simulink library "lib_energy_storage"  (Simulink 7.9)
settings: Solver=ode45  SolverMode=SingleTasking  StartTime=0.0  StopTime=10.0  RelTol=1e-3
undefined symbols (not defined in the file or in its folder): air_cp, amb_tmp, cyc_mph, enable_stop, ess_cap, ess_cap_scale, ess_cb, ess_cc, ess_coulombic_eff, ess_init_soc, ess_max_ah_cap, ess_max_p, ess_max_p_soc, ess_max_soc, ess_max_volts, ess_min_soc, ess_min_volts, ess_MMi, ess_MMo, ess_mod_airflow, ess_mod_cp, ess_mod_cpm, ess_mod_init_tmp, ess_module_mass, ess_module_num, ess_on, ess_parallel_mod_num, ess_r, ess_r_chg, ess_r_dis, ess_rc, ess_re, ess_res_scale_coef, ess_res_scale_fun, ess_rt, ess_set_tmp, ess_soc, ess_th_calc, ess_th_res, ess_th_res_off, ess_th_res_on, ess_tmp, ess_voc, fund_byu, fund_byuop, mc_min_volts, saber_air_temp, Saber_Battery_IO_File, saber_init_soc, saber_init_temp, saber_init_voc, saber_k_cb, saber_k_cc, saber_k_rc, saber_k_re, saber_k_rt, saber_k_soc, t_soc, time_step
libraries: lib_energy_storage x3
(part 3 of 3)

== system lib_energy_storage/Ess Choices/energy storage <ess> optima fundamental model/ess tmp/Tair,ave ==
  Qess_case : Inport
  Enable : EnablePort  StatesWhenEnabling=reset
  Block NOTES : Subsystem
      mask Display: disp('Block\nNOTES')
  Tamb-(Q/mcp)/2 : Fcn  Expr=amb_tmp - (u(1)/(ess_mod_airflow*air_cp))/2
  do ex calcs?1 : Constant  Value=ess_th_res_on
  Tair_ave : Outport  OutputWhenDisabled=reset  InitialOutput=amb_tmp
  Th Res : Outport  Port=2  OutputWhenDisabled=reset  InitialOutput=ess_th_res_off
  wires:
  do ex calcs?1/1 -> Th Res/1
  Qess_case/1 -> Tamb-(Q/mcp)/2/1
  Tamb-(Q/mcp)/2/1 -> Tair_ave/1

== system lib_energy_storage/Ess Choices/Ultracapacitor  System/Calc Iout/limit power/Limits ==
  current req : Inport
  current bat limited : Inport  Port=2
  V used : Inport  Port=3
  V mc_min_volts : Inport  Port=4
  V battery (.5Voc) : Inport  Port=5
  V ess_min_volts : Inport  Port=6
  Relational Operator1 : RelationalOperator  Operator===  InputSameDT=on
  Relational Operator3 : RelationalOperator  Operator===  InputSameDT=on
  Relational Operator4 : RelationalOperator  Operator===  InputSameDT=on
  Relational Operator5 : RelationalOperator  Operator=<=  InputSameDT=on
  limited by battery : Logic
  limited by battery min V : Logic
  limited by motor controller : Logic
  tag scope: ess_minV_limited=global, ess_pwr_limited=global, mc_voltage_limited=global
  wires:
  current bat limited/1 -> Relational Operator1/2
  V mc_min_volts/1 -> Relational Operator3/2
  V used/1 -> Relational Operator3/1, Relational Operator4/1, Relational Operator5/1
  V battery (.5Voc)/1 -> Relational Operator4/2
  V ess_min_volts/1 -> Relational Operator5/2
  limited by motor controller/1 -> [mc_voltage_limited]
  limited by battery/1 -> [ess_pwr_limited]
  limited by battery min V/1 -> [ess_minV_limited]
  Relational Operator3/1 -> limited by motor controller/2
  Relational Operator1/1 -> limited by motor controller/1, limited by battery/1, limited by battery min V/1
  Relational Operator4/1 -> limited by battery/2
  Relational Operator5/1 -> limited by battery min V/2
  current req/1 -> Relational Operator1/1

== system lib_energy_storage/Ess Choices/Ultracapacitor  System/ess tmp/Tair,ave/Block NOTES ==
  note: This block determins the average temperature of the cooling air over the module.

== system lib_energy_storage/Ess Choices/energy storage <ess>/ess tmp/Tair,ave/Block NOTES ==
  note: This block determins the average temperature of the cooling air over the module.

== system lib_energy_storage/Ess Choices/energy storage <ess> RC/Thermal Model of Battery/Tair,ave/Block NOTES ==
  note: This block determins the average temperature of the cooling air over the module.

== system lib_energy_storage/Ess Choices/energy storage <ess> nnet/NNet/Neural Network/Layer 1 ==
  "p{1}" : Inport  PortDimensions=2
  Delays 1 : Subsystem
      mask Display: disp('TDL')
  "IW{1,1}" : Subsystem
      mask Display: disp('weight')
  "b{1}" : Constant  Value=[-6.0348629999999996;2.0410720000000002;2.002373]
      mask Display: disp('bias')
  logsig : Subsystem
      mask Display: plot([-1 1],[0 0],[-1 -.9 -.8 -.7 -.6 -.5 -.4 -.3 -.2 -.1 0 .1 .2 .3 .4 .5 .6 .7 .8 .9 1],1./(1+exp(-8*[-1 -.9 -.8 -.7 -.6 -.5 -.4 -.3 -.2 -.1 0 .1 .2 .3 .4 .5 .6 .7 .8 .9 1]))+.01)
  netsum : Sum  Inputs=2  SaturateOnIntegerOverflow=on  InputSameDT=on  OutDataTypeStr=Inherit: Same as first input
      mask Display: disp('+')
  "a{1}" : Outport  InitialOutput=[0;0;0]
  wires:
  logsig/1(a) -> "a{1}"/1
  netsum/1 -> logsig/1(n)
  "b{1}"/1 -> netsum/2
  "IW{1,1}"/1("iz{1,1}") -> netsum/1
  Delays 1/1("pd{1,1}") -> "IW{1,1}"/1("pd{1,1}")
  "p{1}"/1 -> Delays 1/1("p{1}")

== system lib_energy_storage/Ess Choices/energy storage <ess> nnet/NNet/Neural Network/Layer 2 ==
  "a{1} " : Inport  PortDimensions=3
  Delays 1 : Subsystem
      mask Display: disp('TDL')
  "LW{2,1}" : Subsystem
      mask Display: disp('weight')
  "b{2}" : Constant  Value=[3.0652170000000001;-2.2814760000000001]
      mask Display: disp('bias')
  logsig : Subsystem
      mask Display: plot([-1 1],[0 0],[-1 -.9 -.8 -.7 -.6 -.5 -.4 -.3 -.2 -.1 0 .1 .2 .3 .4 .5 .6 .7 .8 .9 1],1./(1+exp(-8*[-1 -.9 -.8 -.7 -.6 -.5 -.4 -.3 -.2 -.1 0 .1 .2 .3 .4 .5 .6 .7 .8 .9 1]))+.01)
  netsum : Sum  Inputs=2  SaturateOnIntegerOverflow=on  InputSameDT=on  OutDataTypeStr=Inherit: Same as first input
      mask Display: disp('+')
  "a{2}" : Outport  InitialOutput=[0;0]
  wires:
  logsig/1(a) -> "a{2}"/1
  netsum/1 -> logsig/1(n)
  "b{2}"/1 -> netsum/2
  "LW{2,1}"/1("lz{2,1}") -> netsum/1
  Delays 1/1("pd{2,1}") -> "LW{2,1}"/1("ad{2,1}")
  "a{1} "/1 -> Delays 1/1("p{2}")

== system lib_energy_storage/Ess Choices/energy storage <ess> fundamental model/ess tmp/Tair,ave/Block NOTES ==
  note: This block determins the average temperature of the cooling air over the module.

== system lib_energy_storage/Ess Choices/energy storage <ess> optima fundamental model/ess tmp/Tair,ave/Block NOTES ==
  note: This block determins the average temperature of the cooling air over the module.

== system lib_energy_storage/Ess Choices/energy storage <ess> nnet/NNet/Neural Network/Layer 1/Delays 1 ==
  "p{1}" : Inport  PortDimensions=2
  mux : Mux  Inputs=1
  "pd{1,1}" : Outport  InitialOutput=0
  wires:
  mux/1 -> "pd{1,1}"/1
  "p{1}"/1 -> mux/1

== system lib_energy_storage/Ess Choices/energy storage <ess> nnet/NNet/Neural Network/Layer 1/IW{1,1} ==
  "pd{1,1}" : Inport  PortDimensions=2
  "IW{1,1}(1,:)'" : Constant  Value=[-4.5598890000000001;5.793647]
      mask Display: disp('weights')
  "IW{1,1}(2,:)'" : Constant  Value=[-2.8283469999999999;1.417519]
      mask Display: disp('weights')
  "IW{1,1}(3,:)'" : Constant  Value=[-2.3043559999999998;-1.4467429999999999]
      mask Display: disp('weights')
  Mux : Mux  Inputs=3
  dotprod1 : Subsystem
  dotprod2 : Subsystem
  dotprod3 : Subsystem
  "iz{1,1}" : Outport  InitialOutput=0
  wires:
  Mux/1 -> "iz{1,1}"/1
  dotprod3/1(z) -> Mux/3
  "IW{1,1}(3,:)'"/1 -> dotprod3/1(w)
  dotprod2/1(z) -> Mux/2
  "pd{1,1}"/1 -> dotprod3/2(p), dotprod2/2(p), dotprod1/2(p)
  "IW{1,1}(2,:)'"/1 -> dotprod2/1(w)
  dotprod1/1(z) -> Mux/1
  "IW{1,1}(1,:)'"/1 -> dotprod1/1(w)

== system lib_energy_storage/Ess Choices/energy storage <ess> nnet/NNet/Neural Network/Layer 1/logsig ==
  n : Inport
  Exp : ElementaryMath  Operator=exp
  Gain : Gain  Gain=-1  SaturateOnIntegerOverflow=on  OutDataTypeStr=Inherit: Same as input  ParamDataTypeStr=Inherit: Same as input
  Reciprocal : ElementaryMath  Operator=reciprocal
  Sum : Sum  SaturateOnIntegerOverflow=on  InputSameDT=on  OutDataTypeStr=Inherit: Same as first input
  one : Constant
  a : Outport  InitialOutput=0
  wires:
  n/1 -> Gain/1
  Gain/1 -> Exp/1
  Exp/1 -> Sum/1
  one/1 -> Sum/2
  Sum/1 -> Reciprocal/1
  Reciprocal/1 -> a/1

== system lib_energy_storage/Ess Choices/energy storage <ess> nnet/NNet/Neural Network/Layer 2/Delays 1 ==
  "p{2}" : Inport  PortDimensions=3
  mux : Mux  Inputs=1
  "pd{2,1}" : Outport  InitialOutput=0
  wires:
  mux/1 -> "pd{2,1}"/1
  "p{2}"/1 -> mux/1

== system lib_energy_storage/Ess Choices/energy storage <ess> nnet/NNet/Neural Network/Layer 2/LW{2,1} ==
  "ad{2,1}" : Inport  PortDimensions=3
  "IW{2,1}(1,:)'" : Constant  Value=[-0.2776092;-2.6799360000000001;-2.2138360000000001]
      mask Display: disp('weights')
  "IW{2,1}(2,:)'" : Constant  Value=[3.601111;2.064257;0.86618079999999997]
      mask Display: disp('weights')
  Mux : Mux  Inputs=2
  dotprod1 : Subsystem
  dotprod2 : Subsystem
  "lz{2,1}" : Outport  InitialOutput=0
  wires:
  Mux/1 -> "lz{2,1}"/1
  dotprod2/1(z) -> Mux/2
  "ad{2,1}"/1 -> dotprod2/2(p), dotprod1/2(p)
  "IW{2,1}(2,:)'"/1 -> dotprod2/1(w)
  dotprod1/1(z) -> Mux/1
  "IW{2,1}(1,:)'"/1 -> dotprod1/1(w)

== system lib_energy_storage/Ess Choices/energy storage <ess> nnet/NNet/Neural Network/Layer 2/logsig ==
  n : Inport
  Exp : ElementaryMath  Operator=exp
  Gain : Gain  Gain=-1  SaturateOnIntegerOverflow=on  OutDataTypeStr=Inherit: Same as input  ParamDataTypeStr=Inherit: Same as input
  Reciprocal : ElementaryMath  Operator=reciprocal
  Sum : Sum  SaturateOnIntegerOverflow=on  InputSameDT=on  OutDataTypeStr=Inherit: Same as first input
  one : Constant
  a : Outport  InitialOutput=0
  wires:
  n/1 -> Gain/1
  Gain/1 -> Exp/1
  Exp/1 -> Sum/1
  one/1 -> Sum/2
  Sum/1 -> Reciprocal/1
  Reciprocal/1 -> a/1

== system lib_energy_storage/Ess Choices/energy storage <ess> nnet/NNet/Neural Network/Layer 1/IW{1,1}/dotprod1 ==
  w : Inport
  p : Inport  Port=2
  Dot Product : Subsystem  mask(Dot Product){}
      mask help:
      | Inner (dot) product.
      | y=sum(u1.*u2)
      mask init:
      | t=(0:.1:2*pi)';
      | x=cos(t);
      | y=sin(t);
      mask Help: Computes the inner (dot) product of the inputs: sum(u1.*u2).  The inputs are vectors of the same length. Output is a scalar.
      mask Display: plot(0,0,1,1,x*[0.025 0.07]+0.5,y*[0.025 0.07]+0.5)
  z : Outport  InitialOutput=0
  wires:
  w/1 -> Dot Product/1(in_1)
  p/1 -> Dot Product/2(in_2)
  Dot Product/1(out_1) -> z/1

== system lib_energy_storage/Ess Choices/energy storage <ess> nnet/NNet/Neural Network/Layer 1/IW{1,1}/dotprod2 ==
  w : Inport
  p : Inport  Port=2
  Dot Product : Subsystem  mask(Dot Product){}
      mask help:
      | Inner (dot) product.
      | y=sum(u1.*u2)
      mask init:
      | t=(0:.1:2*pi)';
      | x=cos(t);
      | y=sin(t);
      mask Help: Computes the inner (dot) product of the inputs: sum(u1.*u2).  The inputs are vectors of the same length. Output is a scalar.
      mask Display: plot(0,0,1,1,x*[0.025 0.07]+0.5,y*[0.025 0.07]+0.5)
  z : Outport  InitialOutput=0
  wires:
  w/1 -> Dot Product/1(in_1)
  p/1 -> Dot Product/2(in_2)
  Dot Product/1(out_1) -> z/1

== system lib_energy_storage/Ess Choices/energy storage <ess> nnet/NNet/Neural Network/Layer 1/IW{1,1}/dotprod3 ==
  w : Inport
  p : Inport  Port=2
  Dot Product : Subsystem  mask(Dot Product){}
      mask help:
      | Inner (dot) product.
      | y=sum(u1.*u2)
      mask init:
      | t=(0:.1:2*pi)';
      | x=cos(t);
      | y=sin(t);
      mask Help: Computes the inner (dot) product of the inputs: sum(u1.*u2).  The inputs are vectors of the same length. Output is a scalar.
      mask Display: plot(0,0,1,1,x*[0.025 0.07]+0.5,y*[0.025 0.07]+0.5)
  z : Outport  InitialOutput=0
  wires:
  w/1 -> Dot Product/1(in_1)
  p/1 -> Dot Product/2(in_2)
  Dot Product/1(out_1) -> z/1

== system lib_energy_storage/Ess Choices/energy storage <ess> nnet/NNet/Neural Network/Layer 2/LW{2,1}/dotprod1 ==
  w : Inport
  p : Inport  Port=2
  Dot Product : Subsystem  mask(Dot Product){}
      mask help:
      | Inner (dot) product.
      | y=sum(u1.*u2)
      mask init:
      | t=(0:.1:2*pi)';
      | x=cos(t);
      | y=sin(t);
      mask Help: Computes the inner (dot) product of the inputs: sum(u1.*u2).  The inputs are vectors of the same length. Output is a scalar.
      mask Display: plot(0,0,1,1,x*[0.025 0.07]+0.5,y*[0.025 0.07]+0.5)
  z : Outport  InitialOutput=0
  wires:
  w/1 -> Dot Product/1(in_1)
  p/1 -> Dot Product/2(in_2)
  Dot Product/1(out_1) -> z/1

== system lib_energy_storage/Ess Choices/energy storage <ess> nnet/NNet/Neural Network/Layer 2/LW{2,1}/dotprod2 ==
  w : Inport
  p : Inport  Port=2
  Dot Product : Subsystem  mask(Dot Product){}
      mask help:
      | Inner (dot) product.
      | y=sum(u1.*u2)
      mask init:
      | t=(0:.1:2*pi)';
      | x=cos(t);
      | y=sin(t);
      mask Help: Computes the inner (dot) product of the inputs: sum(u1.*u2).  The inputs are vectors of the same length. Output is a scalar.
      mask Display: plot(0,0,1,1,x*[0.025 0.07]+0.5,y*[0.025 0.07]+0.5)
  z : Outport  InitialOutput=0
  wires:
  w/1 -> Dot Product/1(in_1)
  p/1 -> Dot Product/2(in_2)
  Dot Product/1(out_1) -> z/1

== system lib_energy_storage/Ess Choices/energy storage <ess> nnet/NNet/Neural Network/Layer 1/IW{1,1}/dotprod1/Dot Product ==
  in_1 : Inport
  in_2 : Inport  Port=2
  Product : Product  SaturateOnIntegerOverflow=on  RndMeth=Zero  InputSameDT=on  OutDataTypeStr=Inherit: Same as first input
  Sum : Sum  Inputs=+  SaturateOnIntegerOverflow=on  InputSameDT=on  OutDataTypeStr=Inherit: Same as first input
  out_1 : Outport  InitialOutput=0
  wires:
  in_2/1 -> Product/2
  in_1/1 -> Product/1
  Product/1 -> Sum/1
  Sum/1 -> out_1/1

== system lib_energy_storage/Ess Choices/energy storage <ess> nnet/NNet/Neural Network/Layer 1/IW{1,1}/dotprod2/Dot Product ==
  in_1 : Inport
  in_2 : Inport  Port=2
  Product : Product  SaturateOnIntegerOverflow=on  RndMeth=Zero  InputSameDT=on  OutDataTypeStr=Inherit: Same as first input
  Sum : Sum  Inputs=+  SaturateOnIntegerOverflow=on  InputSameDT=on  OutDataTypeStr=Inherit: Same as first input
  out_1 : Outport  InitialOutput=0
  wires:
  in_2/1 -> Product/2
  in_1/1 -> Product/1
  Product/1 -> Sum/1
  Sum/1 -> out_1/1

== system lib_energy_storage/Ess Choices/energy storage <ess> nnet/NNet/Neural Network/Layer 1/IW{1,1}/dotprod3/Dot Product ==
  in_1 : Inport
  in_2 : Inport  Port=2
  Product : Product  SaturateOnIntegerOverflow=on  RndMeth=Zero  InputSameDT=on  OutDataTypeStr=Inherit: Same as first input
  Sum : Sum  Inputs=+  SaturateOnIntegerOverflow=on  InputSameDT=on  OutDataTypeStr=Inherit: Same as first input
  out_1 : Outport  InitialOutput=0
  wires:
  in_2/1 -> Product/2
  in_1/1 -> Product/1
  Product/1 -> Sum/1
  Sum/1 -> out_1/1

== system lib_energy_storage/Ess Choices/energy storage <ess> nnet/NNet/Neural Network/Layer 2/LW{2,1}/dotprod1/Dot Product ==
  in_1 : Inport
  in_2 : Inport  Port=2
  Product : Product  SaturateOnIntegerOverflow=on  RndMeth=Zero  InputSameDT=on  OutDataTypeStr=Inherit: Same as first input
  Sum : Sum  Inputs=+  SaturateOnIntegerOverflow=on  InputSameDT=on  OutDataTypeStr=Inherit: Same as first input
  out_1 : Outport  InitialOutput=0
  wires:
  in_2/1 -> Product/2
  in_1/1 -> Product/1
  Product/1 -> Sum/1
  Sum/1 -> out_1/1

== system lib_energy_storage/Ess Choices/energy storage <ess> nnet/NNet/Neural Network/Layer 2/LW{2,1}/dotprod2/Dot Product ==
  in_1 : Inport
  in_2 : Inport  Port=2
  Product : Product  SaturateOnIntegerOverflow=on  RndMeth=Zero  InputSameDT=on  OutDataTypeStr=Inherit: Same as first input
  Sum : Sum  Inputs=+  SaturateOnIntegerOverflow=on  InputSameDT=on  OutDataTypeStr=Inherit: Same as first input
  out_1 : Outport  InitialOutput=0
  wires:
  in_2/1 -> Product/2
  in_1/1 -> Product/1
  Product/1 -> Sum/1
  Sum/1 -> out_1/1
